simulink library "utils"  (Simulink 9.1)
settings: Solver=VariableStepAuto  StartTime=0.0  StopTime=10.0  RelTol=1e-3
undefined symbols (not defined in the file): DiscIntNeverNeededParam, model_sample_time
libraries: $bdroot x7, simulink_need_slupdate x1
settings Model: SuppressorTable=22 serialization::archive 11 0 6 0 0 0 1 0  Creator=lars  LastModifiedBy=lars

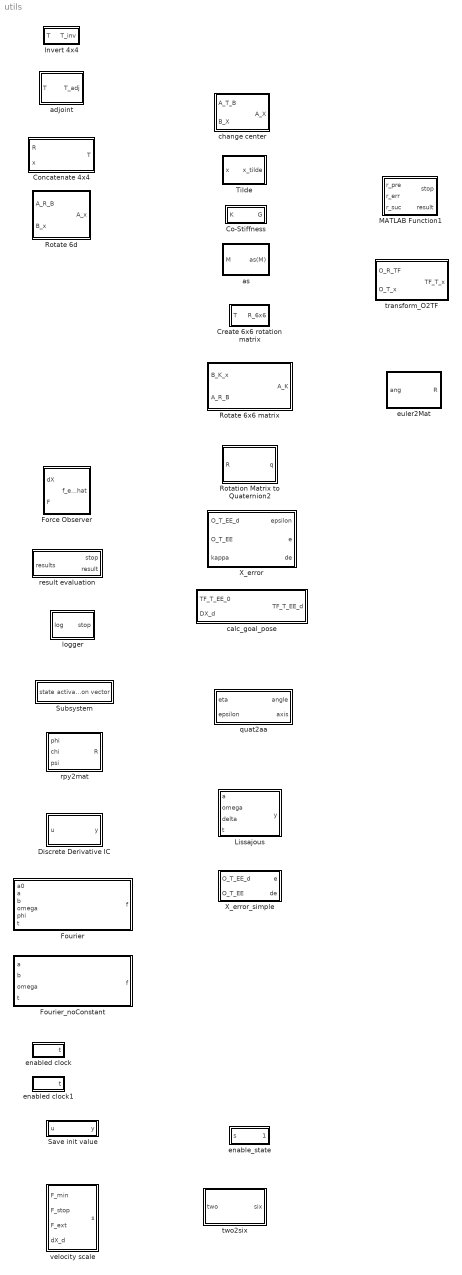
== system utils ==
  Co-Stiffness : Subsystem
  Concatenate 4x4 : Subsystem
  Create 6x6 rotation matrix : Subsystem
  Discrete Derivative IC : Subsystem  mask{model_sample_time=model_sample_time}
      mask prompts: model_sample_time "Sample Time"
  Force Observer : Subsystem
  Fourier : MATLAB Function  TreatAsAtomicUnit=on
  Fourier_noConstant : MATLAB Function  TreatAsAtomicUnit=on
  Invert 4x4 : Subsystem
  Lissajous : MATLAB Function  TreatAsAtomicUnit=on
  MATLAB Function1 : MATLAB Function  TreatAsAtomicUnit=on
  Rotate 6d : Subsystem
  Rotate 6x6 matrix : Subsystem
  Rotation Matrix to Quaternion2 : MATLAB Function  TreatAsAtomicUnit=on
  Save init value : MATLAB Function  TreatAsAtomicUnit=on
  Subsystem : Subsystem  mask{table=[1 0 0;0 1 0;0 0 1]}
      mask prompts: table "State table"
  Tilde : Subsystem
  X_error : Subsystem  TreatAsAtomicUnit=on
  X_error_simple : Subsystem  TreatAsAtomicUnit=on
  adjoint : Subsystem
  as : Subsystem
  calc_goal_pose : MATLAB Function  TreatAsAtomicUnit=on
  change center : Subsystem
  enable_state : Subsystem  mask{valid_state=1}
      mask prompts: valid_state "Valid State"
  enabled clock : Subsystem
  enabled clock1 : Subsystem
  euler2Mat : MATLAB Function  TreatAsAtomicUnit=on
  logger : Subsystem
  quat2aa : Subsystem
  result evaluation : Subsystem
  rpy2mat : MATLAB Function  TreatAsAtomicUnit=on
  transform_O2TF : Subsystem
  two2six : Subsystem
  velocity scale : MATLAB Function  TreatAsAtomicUnit=on

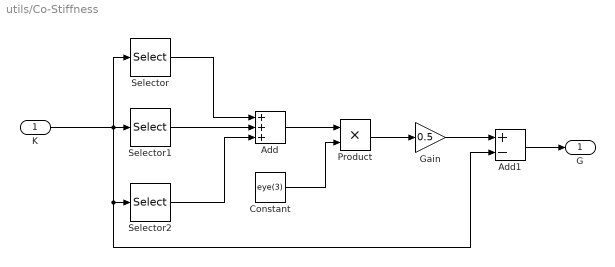
== system utils/Co-Stiffness ==
  K : Inport
  Add : Sum  Inputs=+++
  Add1 : Sum  Inputs=+-
  Constant : Constant  Value=eye(3)
  Gain : Gain  Gain=0.5
  Product : Product
  Selector : Selector  NumberOfDimensions=2  InputPortWidth=3  IndexOptions=Index vector (dialog),Index vector (dialog)  Indices=1,1  OutputSizes=1,1
  Selector1 : Selector  NumberOfDimensions=2  InputPortWidth=3  IndexOptions=Index vector (dialog),Index vector (dialog)  Indices=2,2  OutputSizes=1,1
  Selector2 : Selector  NumberOfDimensions=2  InputPortWidth=3  IndexOptions=Index vector (dialog),Index vector (dialog)  Indices=3,3  OutputSizes=1,1
  G : Outport
  wires:
  K/1 -> Add1/2, Selector2/1, Selector/1, Selector1/1
  Selector/1 -> Add/1
  Selector1/1 -> Add/2
  Selector2/1 -> Add/3
  Add/1 -> Product/1
  Constant/1 -> Product/2
  Product/1 -> Gain/1
  Gain/1 -> Add1/1
  Add1/1 -> G/1

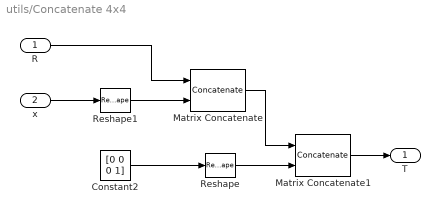
== system utils/Concatenate 4x4 ==
  R : Inport
  x : Inport  Port=2
  Constant2 : Constant  Value=[0 0 0 1]
  Matrix Concatenate : Concatenate  Mode=Multidimensional array  ConcatenateDimension=2
  Matrix Concatenate1 : Concatenate  Mode=Multidimensional array
  Reshape : Reshape  OutputDimensionality=Row vector (2-D)
  Reshape1 : Reshape  OutputDimensionality=Column vector (2-D)
  T : Outport
  wires:
  x/1 -> Reshape1/1
  Constant2/1 -> Reshape/1
  R/1 -> Matrix Concatenate/1
  Matrix Concatenate1/1 -> T/1
  Reshape/1 -> Matrix Concatenate1/2
  Matrix Concatenate/1 -> Matrix Concatenate1/1
  Reshape1/1 -> Matrix Concatenate/2

== system utils/Create 6x6 rotation matrix ==
  T : Inport
  Constant : Constant  Value=zeros(3)
  Matrix Concatenate : Concatenate  Mode=Multidimensional array  ConcatenateDimension=2
  Matrix Concatenate1 : Concatenate  Mode=Multidimensional array  ConcatenateDimension=2
  Matrix Concatenate2 : Concatenate  Mode=Multidimensional array
  Selector : Selector  NumberOfDimensions=2  InputPortWidth=3  IndexOptions=Index vector (dialog),Index vector (dialog)  Indices=1:3,1:3  OutputSizes=1,1
  R_6x6 : Outport
  wires:
  T/1 -> Selector/1
  Selector/1 -> Matrix Concatenate1/2, Matrix Concatenate/1
  Constant/1 -> Matrix Concatenate1/1, Matrix Concatenate/2
  Matrix Concatenate/1 -> Matrix Concatenate2/1
  Matrix Concatenate1/1 -> Matrix Concatenate2/2
  Matrix Concatenate2/1 -> R_6x6/1

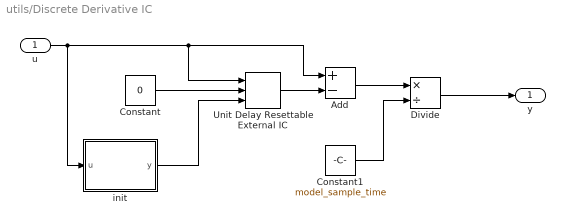
== system utils/Discrete Derivative IC ==
  u : Inport
  Add : Sum  Inputs=+-
  Constant : Constant  Value=0
  Constant1 : Constant  Value=model_sample_time
  Divide : Product  Inputs=*/
  Unit Delay Resettable External IC : simulink_need_slupdate/Unit Delay Resettable External IC  tsamp=-1
      settings: SourceProductName=Simulink  SourceProductBaseCode=SL
  init : MATLAB Function  TreatAsAtomicUnit=on
  y : Outport
  wires:
  Unit Delay Resettable External IC/1 -> Add/2
  u/1 -> init/1(u), Unit Delay Resettable External IC/1, Add/1
  init/1(y) -> Unit Delay Resettable External IC/3
  Constant/1 -> Unit Delay Resettable External IC/2
  Add/1 -> Divide/1
  Divide/1 -> y/1
  Constant1/1 -> Divide/2

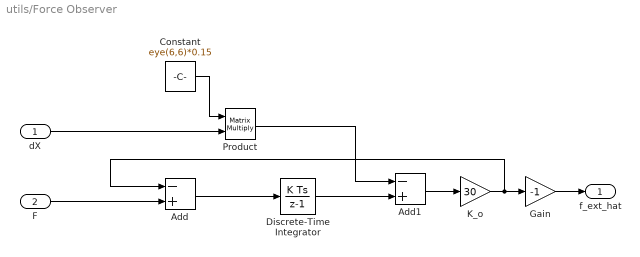
== system utils/Force Observer ==
  dX : Inport
  F : Inport  Port=2
  Add : Sum  Inputs=-+
  Add1 : Sum  Inputs=-+
  Constant : Constant  Value=eye(6,6)*0.15
  Discrete-Time Integrator : DiscreteIntegrator  SampleTime=-1  ICPrevOutput=DiscIntNeverNeededParam  ICPrevScaledInput=DiscIntNeverNeededParam
  Gain : Gain  Gain=-1
  K_o : Gain  Gain=30
  Product : Product  Multiplication=Matrix(*)
  f_ext_hat : Outport
  wires:
  F/1 -> Add/2
  Discrete-Time Integrator/1 -> Add1/2
  Add1/1 -> K_o/1
  Product/1 -> Add1/1
  Add/1 -> Discrete-Time Integrator/1
  dX/1 -> Product/2
  Constant/1 -> Product/1
  K_o/1 -> Add/1, Gain/1
  Gain/1 -> f_ext_hat/1

== system utils/Invert 4x4 ==
  T : Inport
  Concatenate 4x4 : $bdroot/Concatenate 4x4
  Gain : Gain  Gain=-1
  Math Function : Math  Operator=transpose  SaturateOnIntegerOverflow=on
  Product : Product  Multiplication=Matrix(*)
  R : Selector  NumberOfDimensions=2  InputPortWidth=3  IndexOptions=Index vector (dialog),Index vector (dialog)  Indices=1:3,1:3  OutputSizes=1,1
  x : Selector  NumberOfDimensions=2  InputPortWidth=3  IndexOptions=Index vector (dialog),Index vector (dialog)  Indices=1:3,4  OutputSizes=1,1
  T_inv : Outport
  wires:
  T/1 -> x/1, R/1
  R/1 -> Math Function/1
  x/1 -> Product/2
  Product/1 -> Gain/1
  Concatenate 4x4/1 -> T_inv/1
  Math Function/1 -> Concatenate 4x4/1, Product/1
  Gain/1 -> Concatenate 4x4/2

== system utils/Rotate 6d ==
  A_R_B : Inport
  B_x : Inport  Port=2
  Product : Product  Multiplication=Matrix(*)
  Product1 : Product  Multiplication=Matrix(*)
  Select position : Selector  InputPortWidth=6  IndexOptions=Index vector (dialog)  Indices=1:3  OutputSizes=1
  Select rotation : Selector  InputPortWidth=6  IndexOptions=Index vector (dialog)  Indices=4:6  OutputSizes=1
  Vector Concatenate : Concatenate
  A_x : Outport
  wires:
  Product1/1 -> Vector Concatenate/2
  Product/1 -> Vector Concatenate/1
  B_x/1 -> Select position/1, Select rotation/1
  A_R_B/1 -> Product/1, Product1/1
  Vector Concatenate/1 -> A_x/1
  Select position/1 -> Product/2
  Select rotation/1 -> Product1/2

== system utils/Rotate 6x6 matrix ==
  B_K_x : Inport
  A_R_B : Inport  Port=2
  MATLAB Function1 : MATLAB Function  TreatAsAtomicUnit=on
  A_K : Outport
  wires:
  B_K_x/1 -> MATLAB Function1/1(B_K_x)
  A_R_B/1 -> MATLAB Function1/2(A_R_B)
  MATLAB Function1/1(A_K) -> A_K/1

== system utils/Subsystem ==
  state : Inport
  MATLAB Function : MATLAB Function  TreatAsAtomicUnit=on
  table : Constant  Value=table
  activation vector : Outport
  wires:
  state/1 -> MATLAB Function/1(s)
  table/1 -> MATLAB Function/2(table)
  MATLAB Function/1(y) -> activation vector/1

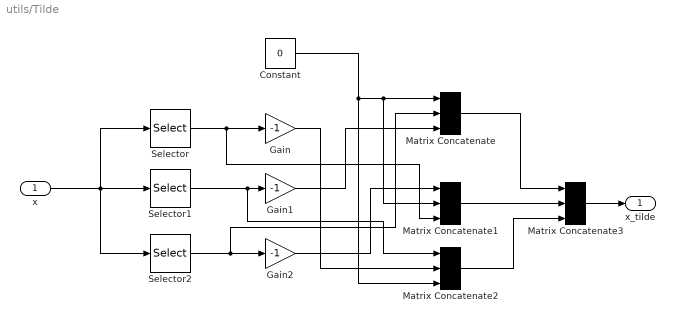
== system utils/Tilde ==
  x : Inport
  Constant : Constant  Value=0
  Gain : Gain  Gain=-1
  Gain1 : Gain  Gain=-1
  Gain2 : Gain  Gain=-1
  Matrix Concatenate : Concatenate  NumInputs=3  Mode=Multidimensional array
  Matrix Concatenate1 : Concatenate  NumInputs=3  Mode=Multidimensional array
  Matrix Concatenate2 : Concatenate  NumInputs=3  Mode=Multidimensional array
  Matrix Concatenate3 : Concatenate  NumInputs=3  Mode=Multidimensional array  ConcatenateDimension=2
  Selector : Selector  InputPortWidth=3  IndexOptions=Index vector (dialog)  Indices=1  OutputSizes=1
  Selector1 : Selector  InputPortWidth=3  IndexOptions=Index vector (dialog)  Indices=2  OutputSizes=1
  Selector2 : Selector  InputPortWidth=3  IndexOptions=Index vector (dialog)  Indices=3  OutputSizes=1
  x_tilde : Outport
  wires:
  Selector/1 -> Matrix Concatenate1/3, Gain/1
  x/1 -> Selector/1, Selector1/1, Selector2/1
  Selector1/1 -> Matrix Concatenate2/1, Gain1/1
  Selector2/1 -> Matrix Concatenate/2, Gain2/1
  Matrix Concatenate1/1 -> Matrix Concatenate3/2
  Matrix Concatenate2/1 -> Matrix Concatenate3/3
  Matrix Concatenate/1 -> Matrix Concatenate3/1
  Matrix Concatenate3/1 -> x_tilde/1
  Constant/1 -> Matrix Concatenate2/3, Matrix Concatenate1/2, Matrix Concatenate/1
  Gain1/1 -> Matrix Concatenate/3
  Gain2/1 -> Matrix Concatenate1/1
  Gain/1 -> Matrix Concatenate2/2

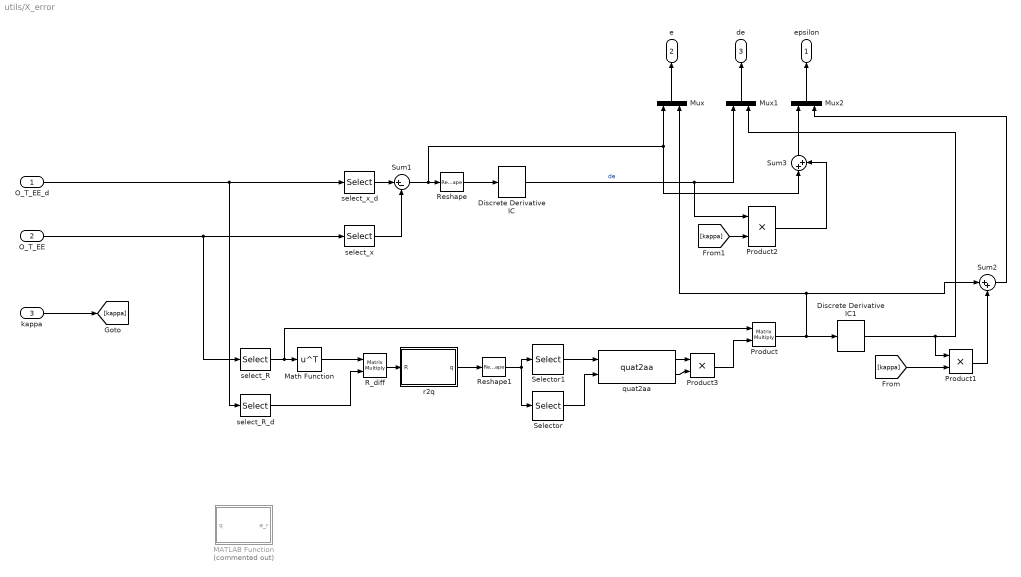
== system utils/X_error ==
  O_T_EE_d : Inport
  O_T_EE : Inport  Port=2
  kappa : Inport  Port=3
  Discrete Derivative IC : $bdroot/Discrete Derivative IC  model_sample_time=model_sample_time
  Discrete Derivative IC1 : $bdroot/Discrete Derivative IC  model_sample_time=model_sample_time
  MATLAB Function : MATLAB Function  Commented=on  TreatAsAtomicUnit=on
  Math Function : Math  Operator=transpose  SaturateOnIntegerOverflow=on
  Mux : Mux  Inputs=2
  Mux1 : Mux  Inputs=2
  Mux2 : Mux  Inputs=2
  Product : Product  Multiplication=Matrix(*)
  Product1 : Product  RndMeth=Zero
  Product2 : Product  RndMeth=Zero
  Product3 : Product
  R_diff : Product  Multiplication=Matrix(*)
  Reshape : Reshape
  Reshape1 : Reshape
  Selector : Selector  InputPortWidth=4  IndexOptions=Index vector (dialog)  Indices=2:4  OutputSizes=1
  Selector1 : Selector  InputPortWidth=4  IndexOptions=Index vector (dialog)  Indices=1  OutputSizes=1
  Sum1 : Sum  Inputs=|+-  SaturateOnIntegerOverflow=on
  Sum2 : Sum  Inputs=|++  SaturateOnIntegerOverflow=on
  Sum3 : Sum  Inputs=|++  SaturateOnIntegerOverflow=on
  quat2aa : $bdroot/quat2aa
  r2q : MATLAB Function  TreatAsAtomicUnit=on
  select_R : Selector  NumberOfDimensions=2  InputPortWidth=3  IndexOptions=Index vector (dialog),Index vector (dialog)  Indices=[1:3],[1:3]  OutputSizes=1,1
  select_R_d : Selector  NumberOfDimensions=2  InputPortWidth=3  IndexOptions=Index vector (dialog),Index vector (dialog)  Indices=[1:3],[1:3]  OutputSizes=1,1
  select_x : Selector  NumberOfDimensions=2  InputPortWidth=3  IndexOptions=Index vector (dialog),Index vector (dialog)  Indices=[1:3],4  OutputSizes=1,1
  select_x_d : Selector  NumberOfDimensions=2  InputPortWidth=3  IndexOptions=Index vector (dialog),Index vector (dialog)  Indices=[1:3],4  OutputSizes=1,1
  epsilon : Outport
  e : Outport  Port=2
  de : Outport  Port=3
  wires:
  quat2aa/2 -> Product3/2
  quat2aa/1 -> Product3/1
  Selector1/1 -> quat2aa/1
  Selector/1 -> quat2aa/2
  kappa/1 -> [kappa]
  Reshape/1 -> Discrete Derivative IC/1
  select_x_d/1 -> Sum1/1
  select_x/1 -> Sum1/2
  Sum1/1 -> Sum3/1, Mux/1, Reshape/1
  [kappa] -> Product2/2
  O_T_EE/1 -> select_R/1, select_x/1
  Discrete Derivative IC/1 -> Product2/1, Mux1/1  "de"
  O_T_EE_d/1 -> select_R_d/1, select_x_d/1
  select_R_d/1 -> R_diff/2
  Product/1 -> Discrete Derivative IC1/1, Sum2/1, Mux/2
  Sum2/1 -> Mux2/2
  Discrete Derivative IC1/1 -> Product1/1, Mux1/2
  R_diff/1 -> r2q/1(R)
  select_R/1 -> Math Function/1, Product/1
  Math Function/1 -> R_diff/1
  r2q/1(q) -> Reshape1/1
  Mux/1 -> e/1
  Mux1/1 -> de/1
  Mux2/1 -> epsilon/1
  Sum3/1 -> Mux2/1
  Reshape1/1 -> Selector1/1, Selector/1
  Product3/1 -> Product/2
  Product2/1 -> Sum3/2
  [kappa] -> Product1/2
  Product1/1 -> Sum2/2

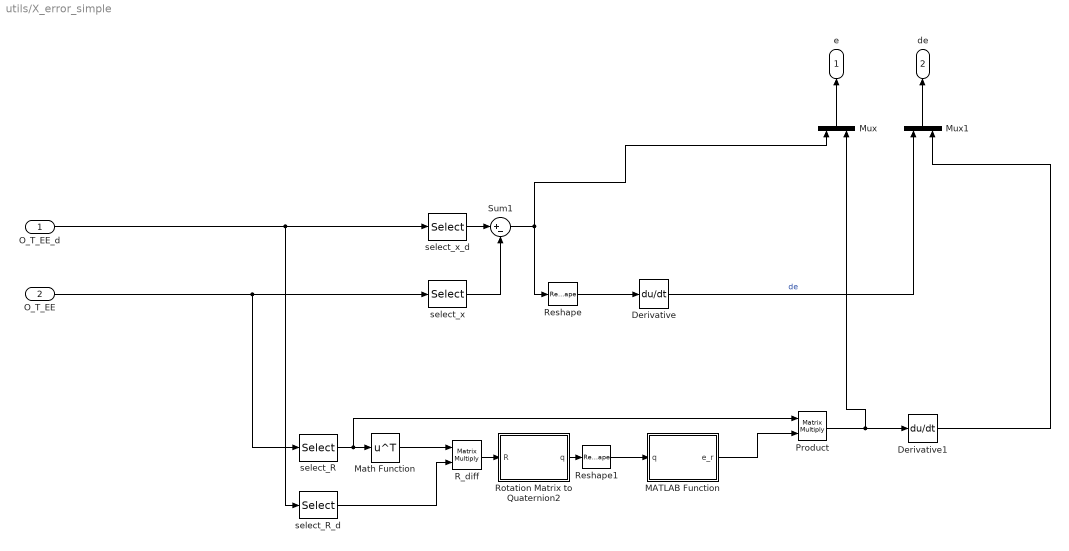
== system utils/X_error_simple ==
  O_T_EE_d : Inport
  O_T_EE : Inport  Port=2
  Derivative : Derivative
  Derivative1 : Derivative
  MATLAB Function : MATLAB Function  TreatAsAtomicUnit=on
  Math Function : Math  Operator=transpose  SaturateOnIntegerOverflow=on
  Mux : Mux  Inputs=2
  Mux1 : Mux  Inputs=2
  Product : Product  Multiplication=Matrix(*)
  R_diff : Product  Multiplication=Matrix(*)
  Reshape : Reshape
  Reshape1 : Reshape
  Rotation Matrix to Quaternion2 : MATLAB Function  TreatAsAtomicUnit=on
  Sum1 : Sum  Inputs=|+-  SaturateOnIntegerOverflow=on
  select_R : Selector  NumberOfDimensions=2  InputPortWidth=3  IndexOptions=Index vector (dialog),Index vector (dialog)  Indices=[1:3],[1:3]  OutputSizes=1,1
  select_R_d : Selector  NumberOfDimensions=2  InputPortWidth=3  IndexOptions=Index vector (dialog),Index vector (dialog)  Indices=[1:3],[1:3]  OutputSizes=1,1
  select_x : Selector  NumberOfDimensions=2  InputPortWidth=3  IndexOptions=Index vector (dialog),Index vector (dialog)  Indices=[1:3],4  OutputSizes=1,1
  select_x_d : Selector  NumberOfDimensions=2  InputPortWidth=3  IndexOptions=Index vector (dialog),Index vector (dialog)  Indices=[1:3],4  OutputSizes=1,1
  e : Outport
  de : Outport  Port=2
  wires:
  MATLAB Function/1(e_r) -> Product/2
  Reshape1/1 -> MATLAB Function/1(q)
  Mux1/1 -> de/1
  Mux/1 -> e/1
  Rotation Matrix to Quaternion2/1(q) -> Reshape1/1
  Math Function/1 -> R_diff/1
  select_R/1 -> Product/1, Math Function/1
  R_diff/1 -> Rotation Matrix to Quaternion2/1(R)
  Derivative1/1 -> Mux1/2
  Product/1 -> Mux/2, Derivative1/1
  select_R_d/1 -> R_diff/2
  O_T_EE_d/1 -> select_x_d/1, select_R_d/1
  Derivative/1 -> Mux1/1  "de"
  O_T_EE/1 -> select_x/1, select_R/1
  select_x/1 -> Sum1/2
  select_x_d/1 -> Sum1/1
  Sum1/1 -> Reshape/1, Mux/1
  Reshape/1 -> Derivative/1

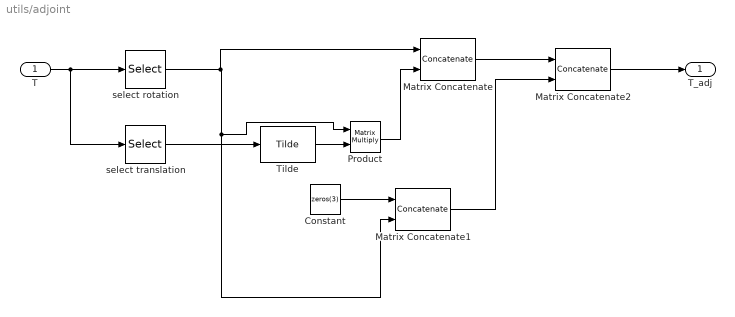
== system utils/adjoint ==
  T : Inport
  Constant : Constant  Value=zeros(3)
  Matrix Concatenate : Concatenate  Mode=Multidimensional array  ConcatenateDimension=2
  Matrix Concatenate1 : Concatenate  Mode=Multidimensional array  ConcatenateDimension=2
  Matrix Concatenate2 : Concatenate  Mode=Multidimensional array
  Product : Product  Multiplication=Matrix(*)
  Tilde : $bdroot/Tilde
  select rotation : Selector  NumberOfDimensions=2  InputPortWidth=3  IndexOptions=Index vector (dialog),Index vector (dialog)  Indices=1:3,1:3  OutputSizes=1,1
  select translation : Selector  NumberOfDimensions=2  InputPortWidth=3  IndexOptions=Index vector (dialog),Index vector (dialog)  Indices=1:3,4  OutputSizes=1,1
  T_adj : Outport
  wires:
  select rotation/1 -> Matrix Concatenate/1, Product/1, Matrix Concatenate1/2
  T/1 -> select translation/1, select rotation/1
  Matrix Concatenate2/1 -> T_adj/1
  Matrix Concatenate/1 -> Matrix Concatenate2/1
  Matrix Concatenate1/1 -> Matrix Concatenate2/2
  Constant/1 -> Matrix Concatenate1/1
  select translation/1 -> Tilde/1
  Tilde/1 -> Product/2
  Product/1 -> Matrix Concatenate/2

== system utils/as ==
  M : Inport
  Add : Sum  Inputs=+-
  Gain : Gain  Gain=0.5
  Math Function : Math  Operator=transpose  SaturateOnIntegerOverflow=on
  as(M) : Outport
  wires:
  M/1 -> Add/1, Math Function/1
  Math Function/1 -> Add/2
  Add/1 -> Gain/1
  Gain/1 -> as(M)/1

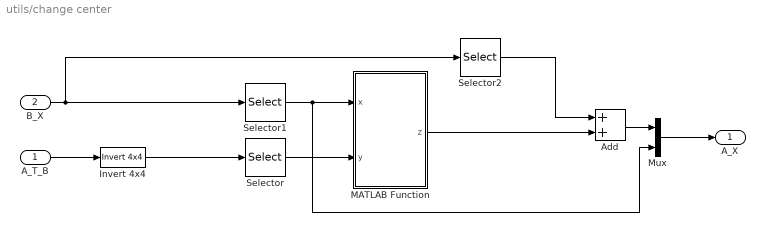
== system utils/change center ==
  A_T_B : Inport
  B_X : Inport  Port=2
  Add : Sum
  Invert 4x4 : $bdroot/Invert 4x4
  MATLAB Function : MATLAB Function  TreatAsAtomicUnit=on
  Mux : Mux  Inputs=2
  Selector : Selector  NumberOfDimensions=2  InputPortWidth=3  IndexOptions=Index vector (dialog),Index vector (dialog)  Indices=1:3,4  OutputSizes=1,1
  Selector1 : Selector  InputPortWidth=6  IndexOptions=Index vector (dialog)  Indices=4:6  OutputSizes=1
  Selector2 : Selector  InputPortWidth=6  IndexOptions=Index vector (dialog)  Indices=1:3  OutputSizes=1
  A_X : Outport
  wires:
  Mux/1 -> A_X/1
  Add/1 -> Mux/1
  Invert 4x4/1 -> Selector/1
  A_T_B/1 -> Invert 4x4/1
  Selector/1 -> MATLAB Function/2(y)
  B_X/1 -> Selector1/1, Selector2/1
  Selector1/1 -> MATLAB Function/1(x), Mux/2
  MATLAB Function/1(z) -> Add/2
  Selector2/1 -> Add/1

== system utils/enable_state ==
  s : Inport
  Constant : Constant  Value=valid_state
  Relational Operator : RelationalOperator  Operator===  OutDataTypeStr=boolean  RndMeth=Simplest
  enable : Outport
  wires:
  Relational Operator/1 -> enable/1
  s/1 -> Relational Operator/1
  Constant/1 -> Relational Operator/2

== system utils/enabled clock ==
  Add : Sum  Inputs=+-
  Digital Clock2 : DigitalClock  SampleTime=model_sample_time
  Hold value : MATLAB Function  TreatAsAtomicUnit=on
  t : Outport
  wires:
  Add/1 -> t/1
  Hold value/1(y) -> Add/2
  Digital Clock2/1 -> Hold value/1(u), Add/1

== system utils/enabled clock1 ==
  Enable : EnablePort
  Add : Sum  Inputs=+-
  Digital Clock2 : DigitalClock  SampleTime=model_sample_time
  Hold value : MATLAB Function  TreatAsAtomicUnit=on
  t : Outport
  wires:
  Digital Clock2/1 -> Add/1, Hold value/1(u)
  Hold value/1(y) -> Add/2
  Add/1 -> t/1

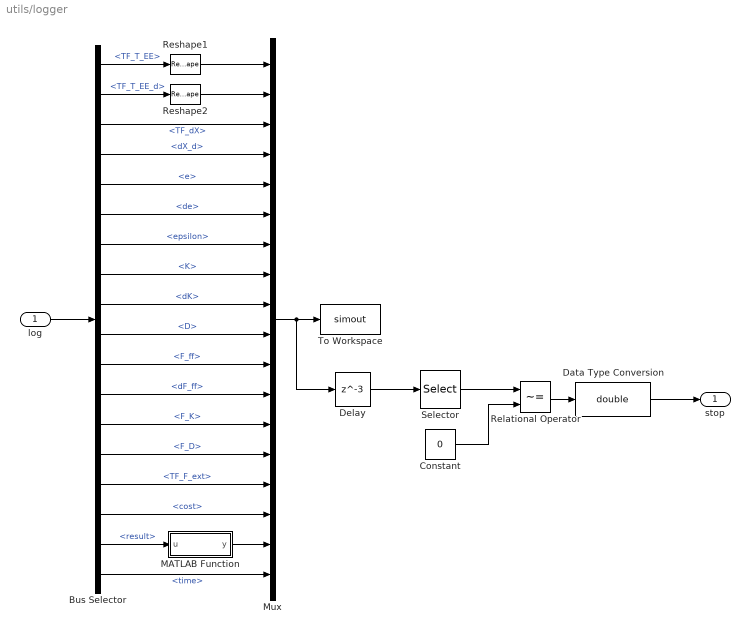
== system utils/logger ==
  log : Inport  OutDataTypeStr=Bus: log_sim
  Bus Selector : BusSelector  OutputSignals=robot.log_percepts.TF_T_EE,robot.interpolator.TF_T_EE_d,robot.log_percepts.TF_dX,robot.interpolator.dX_d,robot.controller.impedance.e,robot.controller.impedance.de,robot.controller.impedance.epsilon,robot.controller.adaptation.stiffness.K,robot.controller.adaptation.stiffness.dK,robot.controller.impedance.D,robot.controller.adaptation.feed_forward.F_ff,robot.controller.adaptation.feed_forward.dF_ff,robot.controller.impedance.F_K,robot.controller.impedance.F_D,robot.log_percepts.TF_F_ext,skill.eval.cost,skill.eval.result,general.time
  Constant : Constant  Value=0
  Data Type Conversion : DataTypeConversion  OutDataTypeStr=double
  Delay : Delay  DelayLength=3
  MATLAB Function : MATLAB Function  TreatAsAtomicUnit=on
  Mux : Mux  Inputs=18
  Relational Operator : RelationalOperator  Operator=~=  OutDataTypeStr=boolean  RndMeth=Simplest
  Reshape1 : Reshape
  Reshape2 : Reshape
  Selector : Selector  InputPortWidth=113  IndexOptions=Index vector (dialog)  Indices=112  OutputSizes=1
  To Workspace : ToWorkspace  VariableName=simout  SaveFormat=Structure With Time  SampleTime=-1
      settings: Priority=100
  stop : Outport  Priority=0
  wires:
  Data Type Conversion/1 -> stop/1
  MATLAB Function/1(y) -> Mux/17
  Delay/1 -> Selector/1
  Mux/1 -> To Workspace/1, Delay/1
  Relational Operator/1 -> Data Type Conversion/1
  Bus Selector/18 -> Mux/18  "<time>"
  Bus Selector/17 -> MATLAB Function/1(u)  "<result>"
  log/1 -> Bus Selector/1
  Bus Selector/2 -> Reshape2/1  "<TF_T_EE_d>"
  Bus Selector/1 -> Reshape1/1  "<TF_T_EE>"
  Reshape1/1 -> Mux/1
  Reshape2/1 -> Mux/2
  Bus Selector/8 -> Mux/8  "<K>"
  Bus Selector/9 -> Mux/9  "<dK>"
  Bus Selector/10 -> Mux/10  "<D>"
  Bus Selector/11 -> Mux/11  "<F_ff>"
  Bus Selector/12 -> Mux/12  "<dF_ff>"
  Bus Selector/13 -> Mux/13  "<F_K>"
  Bus Selector/14 -> Mux/14  "<F_D>"
  Bus Selector/15 -> Mux/15  "<TF_F_ext>"
  Bus Selector/16 -> Mux/16  "<cost>"
  Bus Selector/3 -> Mux/3  "<TF_dX>"
  Bus Selector/4 -> Mux/4  "<dX_d>"
  Bus Selector/5 -> Mux/5  "<e>"
  Bus Selector/6 -> Mux/6  "<de>"
  Bus Selector/7 -> Mux/7  "<epsilon>"
  Selector/1 -> Relational Operator/1
  Constant/1 -> Relational Operator/2

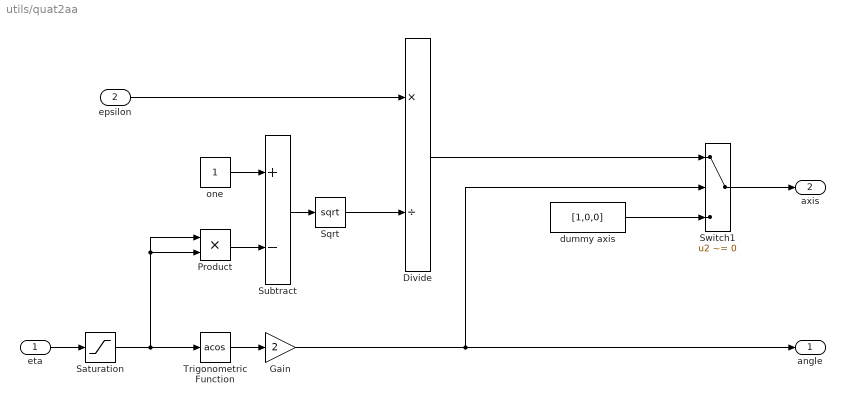
== system utils/quat2aa ==
  eta : Inport
  epsilon : Inport  Port=2
  Divide : Product  Inputs=*/
  Gain : Gain  Gain=2
  Product : Product  RndMeth=Zero
  Saturation : Saturate  UpperLimit=1  LowerLimit=-1
  Sqrt : Sqrt  SaturateOnIntegerOverflow=on
  Subtract : Sum  Inputs=+-
  Switch1 : Switch  Criteria=u2 ~= 0
  Trigonometric Function : Trigonometry  Operator=acos
  dummy axis : Constant  Value=[1,0,0]
  one : Constant
  angle : Outport
  axis : Outport  Port=2
  wires:
  Divide/1 -> Switch1/1
  Switch1/1 -> axis/1
  dummy axis/1 -> Switch1/3
  Gain/1 -> Switch1/2, angle/1
  epsilon/1 -> Divide/1
  Trigonometric Function/1 -> Gain/1
  eta/1 -> Saturation/1
  Subtract/1 -> Sqrt/1
  one/1 -> Subtract/1
  Product/1 -> Subtract/2
  Sqrt/1 -> Divide/2
  Saturation/1 -> Trigonometric Function/1, Product/1, Product/2

== system utils/result evaluation ==
  results : Inport
  Data Type Conversion : DataTypeConversion  OutDataTypeStr=boolean
  MATLAB Function : MATLAB Function  TreatAsAtomicUnit=on
  stop : Outport
  result : Outport  Port=2
  wires:
  MATLAB Function/1(stop) -> Data Type Conversion/1
  results/1 -> MATLAB Function/1(results)
  MATLAB Function/2(result) -> result/1  "result"
  Data Type Conversion/1 -> stop/1  "stop"

== system utils/transform_O2TF ==
  O_R_TF : Inport
  O_T_x : Inport  Port=2
  Concatenate 4x4 : $bdroot/Concatenate 4x4
  Constant : Constant  Value=zeros(3,1)
  Math Function : Math  Operator=transpose  SaturateOnIntegerOverflow=on
  Product : Product  Multiplication=Matrix(*)
  Reshape : Reshape  OutputDimensionality=Customize  OutputDimensions=[4,4]
  TF_T_x : Outport
  wires:
  Reshape/1 -> Product/2
  Constant/1 -> Concatenate 4x4/2
  Concatenate 4x4/1 -> Math Function/1
  O_R_TF/1 -> Concatenate 4x4/1
  O_T_x/1 -> Reshape/1
  Product/1 -> TF_T_x/1
  Math Function/1 -> Product/1

== system utils/two2six ==
  two : Inport
  Demux : Demux  Outputs=2
  Gain : Gain  Gain=[1 1 1]'
  Gain1 : Gain  Gain=[1 1 1]'
  Mux : Mux  Inputs=2
  six : Outport
  wires:
  two/1 -> Demux/1
  Demux/2 -> Gain1/1
  Gain1/1 -> Mux/2
  Demux/1 -> Gain/1
  Gain/1 -> Mux/1
  Mux/1 -> six/1

== matlab function result evaluation/MATLAB Function ==
  data: results input double; stop output double; result output double
function [stop,result] = fcn(results)

result=0;
stop=0;

for i=1:size(results,1)
    if results(i)==1
        result=1;
        stop=1;
        break;
    end
end

for i=1:size(results,1)
    if results(i)==-1
        result=-1;
        stop=1;
        break;
    end
end

== matlab function logger/MATLAB Function ==
  data: u input double; y output double
function y = fcn(u)

persistent flag

if isempty(flag)
    flag=0;
end

if (u==1 || u==-1) && flag==0
    flag=u;
end

y = flag;

== matlab function Rotation Matrix to Quaternion2 ==
  data: R input double; q output double
function q =r2q(R)
%#codegen
q=zeros(1,4);
if ~(all(size(R)==[3,3]))
    error('Bad input dimensions. Input must be 3x3');
end

% Ne dela za specialne kote, ko je s=0 ali v=0
% s=0.5*sqrt(R(1,1)+R(2,2)+R(3,3)+1);
% v=[R(3,2)-R(2,3),R(1,3)-R(3,1),R(2,1)-R(1,2)]'/4/s;
%
% q=quaternion([s v']);

qsx=trace(R)+1;
if qsx>=0
    qs = sqrt(qsx)/2.0;
else
    qs=0;
end
kx = R(3,2) - R(2,3);	% Oz - Ay
ky = R(1,3) - R(3,1);	% Ax - Nz
kz = R(2,1) - R(1,2);	% Ny - Ox

if (R(1,1) >= R(2,2)) && (R(1,1) >= R(3,3))
    kx1 = R(1,1) - R(2,2) - R(3,3) + 1;	% Nx - Oy - Az + 1
    ky1 = R(2,1) + R(1,2);			% Ny + Ox
    kz1 = R(3,1) + R(1,3);			% Nz + Ax
    add = (kx >= 0);
elseif (R(2,2) >= R(3,3))
    kx1 = R(2,1) + R(1,2);			% Ny + Ox
    ky1 = R(2,2) - R(1,1) - R(3,3) + 1;	% Oy - Nx - Az + 1
    kz1 = R(3,2) + R(2,3);			% Oz + Ay
    add = (ky >= 0);
else
    kx1 = R(3,1) + R(1,3);			% Nz + Ax
    ky1 = R(3,2) + R(2,3);			% Oz + Ay
    kz1 = R(3,3) - R(1,1) - R(2,2) + 1;	% Az - Nx - Oy + 1
    add = (kz >= 0);
end

if add
    kx = kx + kx1;
    ky = ky + ky1;
    kz = kz + kz1;
else
    kx = kx - kx1;
    ky = ky - ky1;
    kz = kz - kz1;
end
nm = norm([kx ky kz]);
if nm == 0
    q = [1 0 0 0];
else
    ss=1-qs^2;
    if ss<0
        s=0;
    else
        s = sqrt(ss) / nm;
    end
    qv = s*[kx ky kz];
    
    q = [qs qv];
end

== matlab function change center/MATLAB Function ==
  data: x input double; z output double; y input double
function z = fcn(x,y)

z = cross(x,y);

== matlab function X_error/MATLAB Function ==
  data: q input double; e_r output double
function e_r = fcn(q)

a=sin(acos(complex(q(1))));

a=real(a);

if abs(a)<0.001
    e_r=[0 0 0]';
else
    e_r=[q(2)/a q(3)/a q(4)/a]';
end

== matlab function X_error/r2q ==
  data: R input double; q output double
function q =r2q(R)
%#codegen
q=zeros(1,4);
if ~(all(size(R)==[3,3]))
    error('Bad input dimensions. Input must be 3x3');
end

% Ne dela za specialne kote, ko je s=0 ali v=0
% s=0.5*sqrt(R(1,1)+R(2,2)+R(3,3)+1);
% v=[R(3,2)-R(2,3),R(1,3)-R(3,1),R(2,1)-R(1,2)]'/4/s;
%
% q=quaternion([s v']);

qsx=trace(R)+1;
if qsx>=0
    qs = sqrt(qsx)/2.0;
else
    qs=0;
end
kx = R(3,2) - R(2,3);	% Oz - Ay
ky = R(1,3) - R(3,1);	% Ax - Nz
kz = R(2,1) - R(1,2);	% Ny - Ox

if (R(1,1) >= R(2,2)) && (R(1,1) >= R(3,3))
    kx1 = R(1,1) - R(2,2) - R(3,3) + 1;	% Nx - Oy - Az + 1
    ky1 = R(2,1) + R(1,2);			% Ny + Ox
    kz1 = R(3,1) + R(1,3);			% Nz + Ax
    add = (kx >= 0);
elseif (R(2,2) >= R(3,3))
    kx1 = R(2,1) + R(1,2);			% Ny + Ox
    ky1 = R(2,2) - R(1,1) - R(3,3) + 1;	% Oy - Nx - Az + 1
    kz1 = R(3,2) + R(2,3);			% Oz + Ay
    add = (ky >= 0);
else
    kx1 = R(3,1) + R(1,3);			% Nz + Ax
    ky1 = R(3,2) + R(2,3);			% Oz + Ay
    kz1 = R(3,3) - R(1,1) - R(2,2) + 1;	% Az - Nx - Oy + 1
    add = (kz >= 0);
end

if add
    kx = kx + kx1;
    ky = ky + ky1;
    kz = kz + kz1;
else
    kx = kx - kx1;
    ky = ky - ky1;
    kz = kz - kz1;
end
nm = norm([kx ky kz]);
if nm == 0
    q = [1 0 0 0];
else
    ss=1-qs^2;
    if ss<0
        s=0;
    else
        s = sqrt(ss) / nm;
    end
    qv = s*[kx ky kz];
    
    q = [qs qv];
end

== matlab function Lissajous ==
  data: a input double; y output double; omega input double; delta input double; t input double
function y = fcn(a,omega,delta,t)
y=zeros(length(a),1);
for i=1:length(a)
    y(i)=a(i)*sin(2*pi*omega(i)*t+delta(i));
end

== matlab function calc_goal_pose ==
  data: TF_T_EE_0 input double; TF_T_EE_d output double; DX_d input double
function TF_T_EE_d = fcn(TF_T_EE_0,DX_d)

TF_T_EE_d = TF_T_EE_0;

TF_T_EE_d(1,4) = TF_T_EE_d(1,4)+DX_d(1);
TF_T_EE_d(2,4) = TF_T_EE_d(2,4)+DX_d(2);
TF_T_EE_d(3,4) = TF_T_EE_d(3,4)+DX_d(3);

== matlab function X_error_simple/MATLAB Function ==
  data: q input double; e_r output double
function e_r = fcn(q)

a=sin(acos(complex(q(1))));

a=real(a);

if abs(a)<0.001
    e_r=[0 0 0]';
else
    e_r=[q(2)/a q(3)/a q(4)/a]';
end

== matlab function X_error_simple/Rotation Matrix to Quaternion2 ==
  data: R input double; q output double
function q =r2q(R)
%#codegen
q=zeros(1,4);
if ~(all(size(R)==[3,3]))
    error('Bad input dimensions. Input must be 3x3');
end

% Ne dela za specialne kote, ko je s=0 ali v=0
% s=0.5*sqrt(R(1,1)+R(2,2)+R(3,3)+1);
% v=[R(3,2)-R(2,3),R(1,3)-R(3,1),R(2,1)-R(1,2)]'/4/s;
%
% q=quaternion([s v']);

qsx=trace(R)+1;
if qsx>=0
    qs = sqrt(qsx)/2.0;
else
    qs=0;
end
kx = R(3,2) - R(2,3);	% Oz - Ay
ky = R(1,3) - R(3,1);	% Ax - Nz
kz = R(2,1) - R(1,2);	% Ny - Ox

if (R(1,1) >= R(2,2)) && (R(1,1) >= R(3,3))
    kx1 = R(1,1) - R(2,2) - R(3,3) + 1;	% Nx - Oy - Az + 1
    ky1 = R(2,1) + R(1,2);			% Ny + Ox
    kz1 = R(3,1) + R(1,3);			% Nz + Ax
    add = (kx >= 0);
elseif (R(2,2) >= R(3,3))
    kx1 = R(2,1) + R(1,2);			% Ny + Ox
    ky1 = R(2,2) - R(1,1) - R(3,3) + 1;	% Oy - Nx - Az + 1
    kz1 = R(3,2) + R(2,3);			% Oz + Ay
    add = (ky >= 0);
else
    kx1 = R(3,1) + R(1,3);			% Nz + Ax
    ky1 = R(3,2) + R(2,3);			% Oz + Ay
    kz1 = R(3,3) - R(1,1) - R(2,2) + 1;	% Az - Nx - Oy + 1
    add = (kz >= 0);
end

if add
    kx = kx + kx1;
    ky = ky + ky1;
    kz = kz + kz1;
else
    kx = kx - kx1;
    ky = ky - ky1;
    kz = kz - kz1;
end
nm = norm([kx ky kz]);
if nm == 0
    q = [1 0 0 0];
else
    ss=1-qs^2;
    if ss<0
        s=0;
    else
        s = sqrt(ss) / nm;
    end
    qv = s*[kx ky kz];
    
    q = [qs qv];
end

== matlab function Subsystem/MATLAB Function ==
  data: s input double; y output double; table input double
function y = fcn(s,table)

y = table(s,:);

== matlab function rpy2mat ==
  data: phi input double; R output double; chi input double; psi input double
function R = fcn(phi,chi,psi)

phi=phi/180*pi;
chi=chi/180*pi;
psi=psi/180*pi;

R_psi=[cos(psi) -sin(psi) 0;
    sin(psi) cos(psi) 0;
    0 0 1];

R_chi=[cos(chi) 0 sin(chi);
        0 1 0;
        -sin(chi) 0 cos(chi)];
    
R_phi=[1 0 0;
        0 cos(phi) -sin(phi);
        0 sin(phi) cos(phi)];
    
R=R_psi*R_chi*R_phi;

== matlab function Discrete Derivative IC/init ==
  data: u input double; y output double
function y = fcn(u)
%#codegen

persistent x_0 

if isempty(x_0)
    x_0=u;
end

y = x_0;

== matlab function Fourier ==
  data: a0 input double; a input double; f output double; b input double; omega input double; phi input double; t input double
function f = fcn(a0,a,b,omega,phi,t)

f=zeros(size(a,1),1);
for i=1:size(a,1)
    f(i)=a0(i)/2;
    for j=1:size(a,2)
        f(i)=f(i)+a(i,j)*cos(2*pi*omega(i)*j*t+phi(i))+b(i,j)*sin(2*pi*omega(i)*j*t+phi(i));
    end
end

== matlab function enabled clock/Hold value ==
  data: u input double; y output double
function y = fcn(u)

persistent time

if isempty(time)
    time=u;
end

y = time;

== matlab function Fourier_noConstant ==
  data: a input double; f output double; b input double; omega input double; t input double
function f = fcn(a,b,omega,t)

f=zeros(size(a,1),1);
for i=1:size(a,1)
    for j=1:size(a,2)
        f(i)=f(i)+a(i,j)*cos(2*pi*omega(i)*j*t)+b(i,j)*sin(2*pi*omega(i)*j*t);
    end
end

== matlab function Save init value ==
  data: u input double; y output double
function y = fcn(u)
%#codegen

persistent x_0 

if isempty(x_0)
    x_0=u;
end

y = x_0;

== matlab function MATLAB Function1 ==
  data: stop output double; r_pre input double; result output double; r_err input double; r_suc input double
function [stop,result] = fcn(r_pre,r_err,r_suc)

persistent flag_init

result=0;
stop=0;
if r_pre==0 && isempty(flag_init)
    result=-1;
    stop=1;
elseif r_err==1
    result=-1;
    stop=1;
elseif r_suc==1
    result=1;
    stop=1;
end

if isempty(flag_init)
    flag_init=1;
end

== matlab function euler2Mat ==
  data: ang input double; R output double
function R = fcn(ang)

phi=ang(1)/180*pi;
chi=ang(2)/180*pi;
psi=ang(3)/180*pi;

R_psi=[cos(psi) -sin(psi) 0;
    sin(psi) cos(psi) 0;
    0 0 1];

R_chi=[cos(chi) 0 sin(chi);
        0 1 0;
        -sin(chi) 0 cos(chi)];
    
R_phi=[1 0 0;
        0 cos(phi) -sin(phi);
        0 sin(phi) cos(phi)];
    
R=R_psi*R_chi*R_phi;

== matlab function enabled clock1/Hold value ==
  data: u input double; y output double
function y = fcn(u)

persistent time

if isempty(time)
    time=u;
end

y = time;

== matlab function velocity scale ==
  data: F_min input double; s output double; F_stop input double; F_ext input double; dX_d input double
function s = fcn(F_min,F_stop,F_ext,dX_d)

s=zeros(6,1);
m=zeros(6,1);
c=zeros(6,1);


for i=1:6
    m(i)=-1/(F_stop(i)-F_min(i));
    c(i)=-m(i)*F_stop(i);
    if F_ext(i)*dX_d(i)>0
        s(i)=1;
    else
        if abs(F_ext(i))<F_min(i)
            s(i)=1;
        elseif abs(F_ext(i))<F_stop(i)
            s(i)=m(i)*abs(F_ext(i))+c(i);
        else
            s(i)=-1;
        end
    end
end

for i=1:6
    if(dX_d(i)==0 || F_stop(i)<0)
        s(i)=1;
    end
    if i>3
        s(i)=1;
    end
end

== matlab function Rotate 6x6 matrix/MATLAB Function1 ==
  data: B_K_x input double; A_K output double; A_R_B input double
function A_K = fcn(B_K_x,A_R_B)
%#codegen

B_K=diag(B_K_x);

A_K=[A_R_B*diag(B_K(1:3))*A_R_B' zeros(3);zeros(3) A_R_B*diag(B_K(4:6))*A_R_B'];
